simulink model "LedAccelerometre"  (R2013a)
settings: Solver=FixedStepDiscrete  StartTime=0.0  StopTime=60  FixedStep=0.1  RelTol=1e-3
libraries: ardrone_lib x2
settings Model: Creator=Jon Even ROSENGREN  LastModifiedBy=Arnaud
settings DataIOCC: SignalLoggingSaveFormat=ModelDataLogs
settings OptimizationCC: InitFltsAndDblsToZero=on  OptimizeModelRefInitCode=on  LifeSpan=1
settings DebuggingCC: MultiTaskDSMMsg=warning  MultiTaskCondExecSysMsg=none  StateNameClashWarn=none  StrictBusMsg=None
settings RTWCC: SystemTargetFile=ardrone.tlc  TemplateMakefile=ardrone.tmf  Description=AR.Drone_v2  ProcessScript=ardrone_make_rtw_hook  TargetLang=C++  IncludeERTFirstTime=on
settings CodeAppCC: IgnoreCustomStorageClasses=off
settings STFCustomTargetCC: GenerateSampleERTMain=on  ModelReferenceCompliant=off  CombineOutputUpdateFcns=on  ERTCustomFileBanners=on  SupportContinuousTime=off  SupportNonInlinedSFcns=off  MATLABClassNameForMDSCustomization=Simulink.SoftwareTarget.ERTCustomization  SystemTargetFile=ardrone.tlc
settings ERTTargetCC: ModelReferenceCompliant=off  ParMdlRefBuildCompliant=off  CompOptLevelCompliant=off  ConcurrentExecutionCompliant=off  ERTFirstTimeCompliant=off  ModelStepFunctionPrototypeControlCompliant=off  CPPClassGenCompliant=off  InlinedParameterPlacement=Hierarchical  ERTSrcFileBannerTemplate=example_banner.tlc  ERTHdrFileBannerTemplate=example_banner.tlc  ERTCustomFileTemplate=ardrone_file_process.tlc

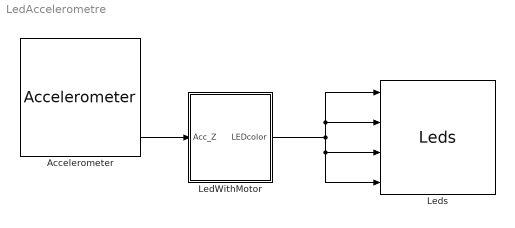
== system LedAccelerometre ==
  Accelerometer : ardrone_lib/Accelerometer  SystemSampleTime=-1
  LedWithMotor : Subsystem
  Leds : ardrone_lib/Leds  SystemSampleTime=-1
  wires:
  Accelerometer/3 -> LedWithMotor/1(Acc_Z)
  LedWithMotor/1(LEDcolor) -> Leds/4, Leds/3, Leds/2, Leds/1

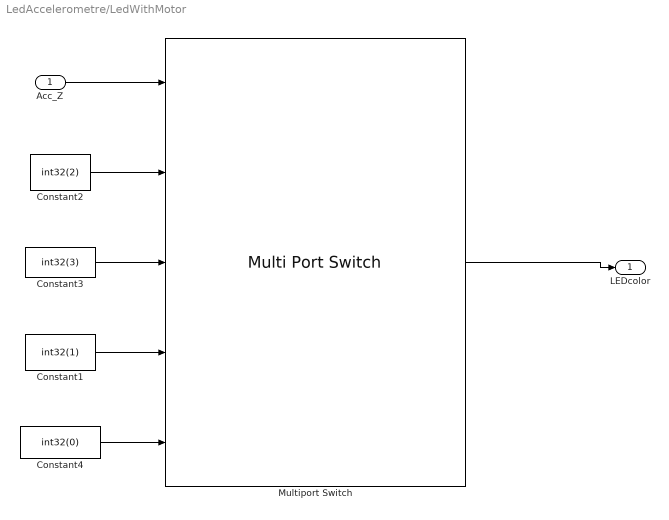
== system LedAccelerometre/LedWithMotor ==
  Acc_Z : Inport
  Constant1 : Constant  Value=int32(1)
  Constant2 : Constant  Value=int32(2)
  Constant3 : Constant  Value=int32(3)
  Constant4 : Constant  Value=int32(0)
  Multiport Switch : MultiPortSwitch  DataPortOrder=Specify indices  Inputs=4  DataPortIndices={[-700:-300],[-299:299],[300:700]}  DataPortForDefault=Additional data port  OutDataTypeStr=int32
  LEDcolor : Outport
  wires:
  Constant2/1 -> Multiport Switch/2
  Constant3/1 -> Multiport Switch/3
  Constant1/1 -> Multiport Switch/4
  Acc_Z/1 -> Multiport Switch/1
  Constant4/1 -> Multiport Switch/5
  Multiport Switch/1 -> LEDcolor/1
